simulink model "tire_normal_loads_model"  (R2023b)
settings: Solver=VariableStepAuto  StartTime=0.0  StopTime=10.0  RelTol=1e-3
undefined symbols (not defined in the file or in its folder): cg_height, front_mass_distribution, g, mass_total, tlltd, track_width_front, track_width_rear, wheelbase
settings Model: Creator=bglen  LastModifiedBy=bglen

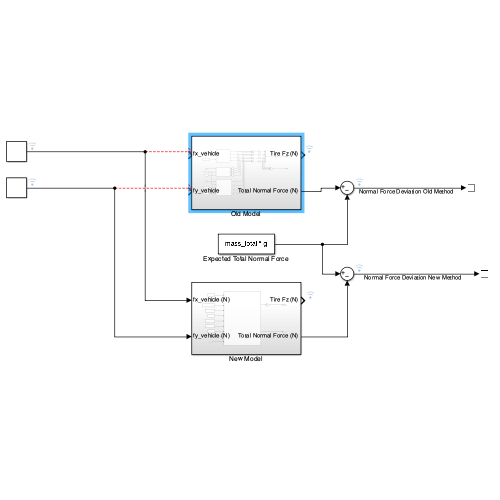
[thumbnail: Simulink's stored preview of the top-level diagram]
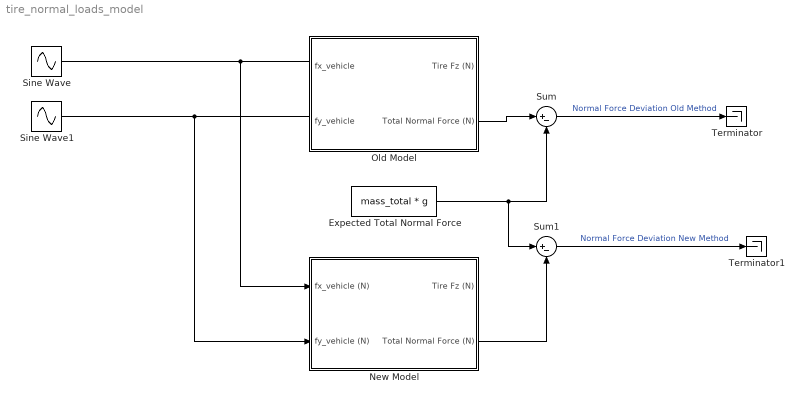
== system tire_normal_loads_model ==
  Expected Total Normal Force : Constant  Value=mass_total * g
  New Model : Subsystem
  Old Model : Subsystem
  Sine Wave : Sin  Amplitude=3000  Frequency=0.5  SampleTime=0
  Sine Wave1 : Sin  Amplitude=3000  Frequency=0.5  SampleTime=0
  Sum : Sum  Inputs=|+-
  Sum1 : Sum  Inputs=|+-
  Terminator : Terminator
  Terminator1 : Terminator
  wires:
  Sine Wave/1 -> New Model/1(fx_vehicle (N))
  Sine Wave1/1 -> New Model/2(fy_vehicle (N))
  Expected Total Normal Force/1 -> Sum/2, Sum1/1
  Old Model/2(Total Normal Force (N)) -> Sum/1
  Sum/1 -> Terminator/1  "Normal Force Deviation Old Method"
  New Model/2(Total Normal Force (N)) -> Sum1/2
  Sum1/1 -> Terminator1/1  "Normal Force Deviation New Method"

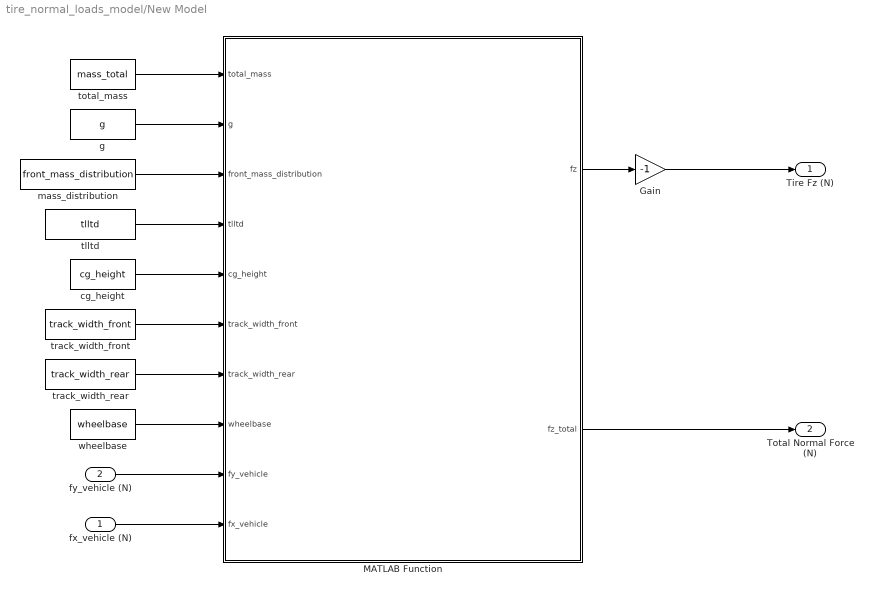
== system tire_normal_loads_model/New Model ==
  fx_vehicle (N) : Inport
  fy_vehicle (N) : Inport  Port=2
  Gain : Gain  Gain=-1
  MATLAB Function : MATLAB Function  TreatAsAtomicUnit=on
  cg_height : Constant  Value=cg_height
  g : Constant  Value=g
  mass_distribution : Constant  Value=front_mass_distribution
  tlltd : Constant  Value=tlltd
  total_mass : Constant  Value=mass_total
  track_width_front : Constant  Value=track_width_front
  track_width_rear : Constant  Value=track_width_rear
  wheelbase : Constant  Value=wheelbase
  Tire Fz (N) : Outport
  Total Normal Force (N) : Outport  Port=2
  wires:
  cg_height/1 -> MATLAB Function/5(cg_height)
  Gain/1 -> Tire Fz (N)/1
  total_mass/1 -> MATLAB Function/1(total_mass)
  mass_distribution/1 -> MATLAB Function/3(front_mass_distribution)
  wheelbase/1 -> MATLAB Function/8(wheelbase)
  tlltd/1 -> MATLAB Function/4(tlltd)
  track_width_front/1 -> MATLAB Function/6(track_width_front)
  track_width_rear/1 -> MATLAB Function/7(track_width_rear)
  fy_vehicle (N)/1 -> MATLAB Function/9(fy_vehicle)
  fx_vehicle (N)/1 -> MATLAB Function/10(fx_vehicle)
  g/1 -> MATLAB Function/2(g)
  MATLAB Function/2(fz_total) -> Total Normal Force (N)/1
  MATLAB Function/1(fz) -> Gain/1

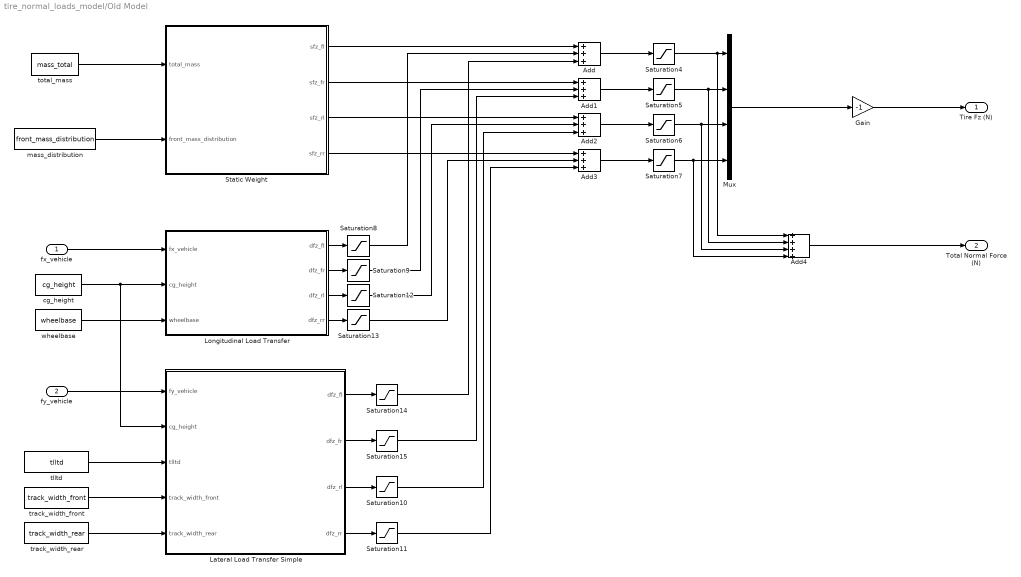
== system tire_normal_loads_model/Old Model ==
  fx_vehicle : Inport
  fy_vehicle : Inport  Port=2
  Add{,1..3} (4 alike) : Sum  Inputs=+++
  Add4 : Sum  Inputs=++++
  Gain : Gain  Gain=-1
  Lateral Load Transfer Simple : MATLAB Function  TreatAsAtomicUnit=on
  Longitudinal Load Transfer : MATLAB Function  TreatAsAtomicUnit=on
  Mux : Mux
  Saturation{8..11,14..15} (6 alike) : Saturate  UpperLimit=(mass_total * front_mass_distribution / 2) * g  LowerLimit=-(mass_total * front_mass_distribution / 2) * g
  Saturation12 : Saturate  UpperLimit=(mass_total * (1 - front_mass_distribution) / 2) * g  LowerLimit=-(mass_total * (1 - front_mass_distribution) / 2) * g
  Saturation13 : Saturate  UpperLimit=(mass_total * (1 - front_mass_distribution) / 2) * g  LowerLimit=-(mass_total * (1 - front_mass_distribution) / 2) * g
  Saturation{4..7} (4 alike) : Saturate  UpperLimit=1000000  LowerLimit=0
  Static Weight : MATLAB Function  TreatAsAtomicUnit=on
  cg_height : Constant  Value=cg_height
  mass_distribution : Constant  Value=front_mass_distribution
  tlltd : Constant  Value=tlltd
  total_mass : Constant  Value=mass_total
  track_width_front : Constant  Value=track_width_front
  track_width_rear : Constant  Value=track_width_rear
  wheelbase : Constant  Value=wheelbase
  Tire Fz (N) : Outport
  Total Normal Force (N) : Outport  Port=2
  wires:
  Saturation6/1 -> Mux/3, Add4/3
  Saturation4/1 -> Mux/1, Add4/1
  Saturation5/1 -> Mux/2, Add4/2
  Mux/1 -> Gain/1
  Saturation7/1 -> Add4/4, Mux/4
  Gain/1 -> Tire Fz (N)/1
  Add4/1 -> Total Normal Force (N)/1
  Lateral Load Transfer Simple/1(dfz_fl) -> Saturation14/1
  Lateral Load Transfer Simple/2(dfz_fr) -> Saturation15/1
  fy_vehicle/1 -> Lateral Load Transfer Simple/1(fy_vehicle)
  Static Weight/4(sfz_rr) -> Add3/1
  Add/1 -> Saturation4/1
  fx_vehicle/1 -> Longitudinal Load Transfer/1(fx_vehicle)
  Add3/1 -> Saturation7/1
  Longitudinal Load Transfer/3(dfz_rl) -> Saturation12/1
  Add1/1 -> Saturation5/1
  Saturation8/1 -> Add/2
  mass_distribution/1 -> Static Weight/2(front_mass_distribution)
  track_width_front/1 -> Lateral Load Transfer Simple/4(track_width_front)
  Longitudinal Load Transfer/2(dfz_fr) -> Saturation9/1
  Static Weight/2(sfz_fr) -> Add1/1
  Static Weight/3(sfz_rl) -> Add2/1
  wheelbase/1 -> Longitudinal Load Transfer/3(wheelbase)
  tlltd/1 -> Lateral Load Transfer Simple/3(tlltd)
  cg_height/1 -> Lateral Load Transfer Simple/2(cg_height), Longitudinal Load Transfer/2(cg_height)
  Lateral Load Transfer Simple/3(dfz_rl) -> Saturation10/1
  Saturation12/1 -> Add2/2
  track_width_rear/1 -> Lateral Load Transfer Simple/5(track_width_rear)
  Longitudinal Load Transfer/4(dfz_rr) -> Saturation13/1
  Saturation14/1 -> Add/3
  Add2/1 -> Saturation6/1
  Lateral Load Transfer Simple/4(dfz_rr) -> Saturation11/1
  Saturation15/1 -> Add1/3
  total_mass/1 -> Static Weight/1(total_mass)
  Saturation13/1 -> Add3/2
  Saturation9/1 -> Add1/2
  Static Weight/1(sfz_fl) -> Add/1
  Longitudinal Load Transfer/1(dfz_fl) -> Saturation8/1
  Saturation10/1 -> Add2/3
  Saturation11/1 -> Add3/3

== matlab function tire_normal_loads_model/New Model/MATLAB Function ==
  data: total_mass input; fz output; g input; front_mass_distribution input; tlltd input; cg_height input; track_width_front input; track_width_rear input; wheelbase input; fy_vehicle input; fx_vehicle input; fz_total output
%{
    
Calculates the normal forces on each tire. It considers the static normal
load, long. load transfer, lateral load transfer using a distribution
constant, and checks for tires lifiting off the ground. It ensures the
total normal load is equal to the vehicle normal force. When multiple tires
are off the ground the load distribution in the grounded tires may be off.
Load transfer from Mx is not implemented.

Note: for aerodynamics add those after this block and not in it.

% Inputs:
% - total_mass: Total mass of the vehicle (kg)
% - g: Gravitational acceleration (m/s^2)
% - static_wd: Static weight distribution as [front, rear]
% - tlltd: Total lateral load transfer distribution (percentage)
% - longitudinal_transfer: Longitudinal load transfer (N)
% - lateral_transfer: Lateral load transfer (N)

Force Directions
when looking from th top of the vehicle:
(+) fx_vehicle is forward
(+) fy_vehicle is to the right

%}

function [fz, fz_total] = normal_loads(total_mass, g, front_mass_distribution, tlltd, cg_height, track_width_front, track_width_rear, wheelbase, fy_vehicle, fx_vehicle)

%% Constants and initial calculations
total_normal_load = total_mass * g; % Total vertical load (N)
static_load_front = front_mass_distribution * total_normal_load;
static_load_rear = (1 - front_mass_distribution) * total_normal_load;
track_width = (track_width_front + track_width_rear) / 2;

%% Static normal loads  as [FL, FR, RL, RR]
Fz_static = [static_load_front / 2, static_load_front / 2, static_load_rear / 2, static_load_rear / 2];

%% Calculate lateral load transfer
% from right tires to left tires
lateral_transfer = (g * fy_vehicle * cg_height) / track_width;
Fz_transfer_lat = lateral_transfer .* [tlltd, -tlltd, (1 - tlltd), -(1 - tlltd)];


%% Calculate longitudinal load transfer
% from front tires to rear tires
longitudinal_transfer = (g * fx_vehicle * cg_height) / wheelbase;
Fz_transfer_long = longitudinal_transfer .* [-1/2, -1/2, 1/2, 1/2];

% Combine static and transfer loads
fz = Fz_static + Fz_transfer_long + Fz_transfer_lat;

%% Clamp negative loads to zero
fz(fz < 0) = 0; % if a tire is off the ground, make it zero so tire model doesnt go crazy

%% Check if redistribution is necessary
% find the tires that are on the ground
grounded_tires = fz > 0;

% Redistribution is needed only if a tire is off the ground
if sum(grounded_tires) < 4

    % correct the other tire normal loads for the contact adjustment
    excess_load = sum(fz) - total_normal_load;
    
    % We will subtract load from tires that are contacting the ground based
    % on the ratios of their normal loads
    fz = fz - (excess_load .* (fz ./ (sum(fz(grounded_tires)))));
end

fz_total = sum(fz);

== matlab function tire_normal_loads_model/Old Model/Lateral Load Transfer Simple ==
  data: dfz_fl output; dfz_fr output; dfz_rl output; dfz_rr output; fy_vehicle input; cg_height input; tlltd input; track_width_front input; track_width_rear input
%{

Calculates lateral load transfer from the vehicle Fy force. Simplified calculation using a constant TLLTD. Units are in
kg, N, m.

Positive Fy is acceleration turning right.

%}
function [dfz_fl, dfz_fr, dfz_rl, dfz_rr] = lateral_load_transfer_simple(fy_vehicle, cg_height, tlltd, track_width_front, track_width_rear)

g = 9.81;

track_width = (track_width_front + track_width_rear) / 2;

% from right tires to left tires
load_transfer = (g * fy_vehicle * cg_height) / track_width;

dfz_fl = load_transfer * tlltd;
dfz_fr = -load_transfer * tlltd;
dfz_rl = load_transfer * (1 - tlltd);
dfz_rr = -load_transfer * (1 - tlltd);

== matlab function tire_normal_loads_model/Old Model/Longitudinal Load Transfer ==
  data: dfz_fl output; dfz_fr output; dfz_rl output; dfz_rr output; fx_vehicle input; cg_height input; wheelbase input
%{

Calculates change in load transfer from the vehicle Fz force. Units are in
kg, N, m.

Positive Fz is acceleration, negative is braking.

%}
function [dfz_fl, dfz_fr, dfz_rl, dfz_rr] = longitudinal_load_transfer(fx_vehicle, cg_height, wheelbase)

g = 9.81;

% from front tires to rear tires
load_transfer = -(g * fx_vehicle * cg_height) / wheelbase;

dfz_fl = load_transfer / 2;
dfz_fr = load_transfer / 2;
dfz_rl = -load_transfer / 2;
dfz_rr = -load_transfer / 2;

== matlab function tire_normal_loads_model/Old Model/Static Weight ==
  data: total_mass input; sfz_fl output; sfz_fr output; sfz_rl output; sfz_rr output; front_mass_distribution input
%{

Calculates static wheel loads. Units are in
kg, N, m.

%}
function [sfz_fl, sfz_fr, sfz_rl, sfz_rr] = static_wheel_load(total_mass, front_mass_distribution)

g = 9.81;

sfz_fl = total_mass * g * front_mass_distribution / 2;
sfz_fr = total_mass * g * front_mass_distribution / 2;
sfz_rl = total_mass * g * (1 - front_mass_distribution) / 2;
sfz_rr = total_mass * g * (1 - front_mass_distribution) / 2;
